simulink model "simulink_model_lab2"  (R2019a)
settings: Solver=VariableStepAuto  StartTime=0.0  StopTime=10.0  RelTol=1e-3
values from neighbouring files (symbols this model uses):
  k = 15    [datafile.m]
settings Model: Creator=abc  LastModifiedBy=abc

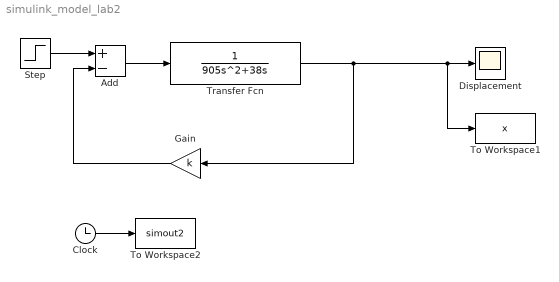
== system simulink_model_lab2 ==
  Add : Sum  Inputs=+-
  Clock : Clock
  Displacement : Scope
  Gain : Gain  Gain=k
  Step : Step  Time=0.1  After=0.02  SampleTime=0
  To Workspace1 : ToWorkspace  VariableName=x  SaveFormat=Timeseries  SampleTime=-1
  To Workspace2 : ToWorkspace  VariableName=simout2  SaveFormat=Timeseries  SampleTime=-1
  Transfer Fcn : TransferFcn  Denominator=[905,38,0]
  wires:
  Add/1 -> Transfer Fcn/1
  Step/1 -> Add/1
  Transfer Fcn/1 -> To Workspace1/1, Displacement/1, Gain/1
  Clock/1 -> To Workspace2/1
  Gain/1 -> Add/2
  ? -> ?
